simulink model "twolinkman"  (R2016a)
settings: Solver=VariableStepAuto  StartTime=0.0  StopTime=10.0  RelTol=1e-4
libraries: simulink x2
settings Model: Creator=Aniket  LastModifiedBy=Aniket

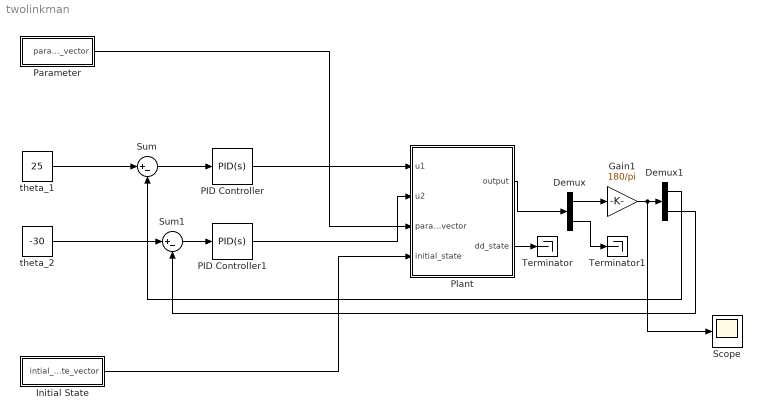
== system twolinkman ==
  Demux : Demux  Outputs=2
  Demux1 : Demux  Outputs=2
  Gain1 : Gain  Gain=180/pi
  Initial State : Subsystem
  PID Controller : simulink/Continuous/PID Controller  Controller=PID  TimeDomain=Continuous-time  SampleTime=-1  IntegratorMethod=Forward Euler  FilterMethod=Forward Euler  Form=Parallel  UseFilter=on  ControllerParametersSource=internal  P=0.928591865622313  I=0.934551024650747  D=0.226303191956831  N=743.239327840978  InitialConditionSource=internal  InitialConditionForIntegrator=0  InitialConditionForFilter=0  ExternalReset=none  LimitOutput=off  UpperSaturationLimit=inf  LowerSaturationLimit=-inf  LinearizeAsGain=on  AntiWindupMode=none  Kb=1  TrackingMode=off  Kt=1  PParamMin=[]  PParamMax=[]  IParamMin=[]  IParamMax=[]  DParamMin=[]  DParamMax=[]  NParamMin=[]  NParamMax=[]  KbParamMin=[]  KbParamMax=[]  KtParamMin=[]  KtParamMax=[]  POutMin=[]  POutMax=[]  IOutMin=[]  IOutMax=[]  DOutMin=[]  DOutMax=[]  NOutMin=[]  NOutMax=[]  KbOutMin=[]  KbOutMax=[]  KtOutMin=[]  KtOutMax=[]  IntegratorOutMin=[]  IntegratorOutMax=[]  FilterOutMin=[]  FilterOutMax=[]  SumOutMin=[]  SumOutMax=[]  SumI1OutMin=[]  SumI1OutMax=[]  SumI2OutMin=[]  SumI2OutMax=[]  SumI3OutMin=[]  SumI3OutMax=[]  SumDOutMin=[]  SumDOutMax=[]  SaturationOutMin=[]  SaturationOutMax=[]  IntegratorContinuousStateAttributes=''  IntegratorStateMustResolveToSignalObject=off  IntegratorRTWStateStorageClass=Auto  FilterContinuousStateAttributes=''  FilterStateMustResolveToSignalObject=off  FilterRTWStateStorageClass=Auto  DifferentiatorICPrevScaledInput=0  DifferentiatorOutMin=[]  DifferentiatorOutMax=[]
  PID Controller1 : simulink/Continuous/PID Controller  Controller=PID  TimeDomain=Continuous-time  SampleTime=-1  IntegratorMethod=Forward Euler  FilterMethod=Forward Euler  Form=Parallel  UseFilter=on  ControllerParametersSource=internal  P=3.82918167781898  I=9.14930088403733  D=0.205650241629809  N=18927.6604658624  InitialConditionSource=internal  InitialConditionForIntegrator=0  InitialConditionForFilter=0  ExternalReset=none  LimitOutput=off  UpperSaturationLimit=inf  LowerSaturationLimit=-inf  LinearizeAsGain=on  AntiWindupMode=none  Kb=1  TrackingMode=off  Kt=1  PParamMin=[]  PParamMax=[]  IParamMin=[]  IParamMax=[]  DParamMin=[]  DParamMax=[]  NParamMin=[]  NParamMax=[]  KbParamMin=[]  KbParamMax=[]  KtParamMin=[]  KtParamMax=[]  POutMin=[]  POutMax=[]  IOutMin=[]  IOutMax=[]  DOutMin=[]  DOutMax=[]  NOutMin=[]  NOutMax=[]  KbOutMin=[]  KbOutMax=[]  KtOutMin=[]  KtOutMax=[]  IntegratorOutMin=[]  IntegratorOutMax=[]  FilterOutMin=[]  FilterOutMax=[]  SumOutMin=[]  SumOutMax=[]  SumI1OutMin=[]  SumI1OutMax=[]  SumI2OutMin=[]  SumI2OutMax=[]  SumI3OutMin=[]  SumI3OutMax=[]  SumDOutMin=[]  SumDOutMax=[]  SaturationOutMin=[]  SaturationOutMax=[]  IntegratorContinuousStateAttributes=''  IntegratorStateMustResolveToSignalObject=off  IntegratorRTWStateStorageClass=Auto  FilterContinuousStateAttributes=''  FilterStateMustResolveToSignalObject=off  FilterRTWStateStorageClass=Auto  DifferentiatorICPrevScaledInput=0  DifferentiatorOutMin=[]  DifferentiatorOutMax=[]
  Parameter : Subsystem
  Plant : Subsystem
  Scope : Scope
  Sum : Sum  Inputs=|+-
  Sum1 : Sum  Inputs=|+-
  Terminator : Terminator
  Terminator1 : Terminator
  theta_1 : Constant  Value=25
  theta_2 : Constant  Value=-30
  wires:
  Plant/1(output) -> Demux/1
  Demux/1 -> Gain1/1
  theta_1/1 -> Sum/1
  theta_2/1 -> Sum1/1
  Sum/1 -> PID Controller/1
  PID Controller/1 -> Plant/1(u1)
  PID Controller1/1 -> Plant/2(u2)
  Sum1/1 -> PID Controller1/1
  Gain1/1 -> Scope/1, Demux1/1
  Demux1/1 -> Sum/2
  Demux1/2 -> Sum1/2
  Parameter/1("param_vector ") -> Plant/3(param_vector)
  Initial State/1(intial_state_vector) -> Plant/4(initial_state)
  Plant/2(dd_state) -> Terminator/1
  Demux/2 -> Terminator1/1

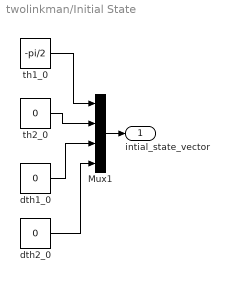
== system twolinkman/Initial State ==
  Mux1 : Mux
  dth1_0 : Constant  Value=0
  dth2_0 : Constant  Value=0
  th1_0 : Constant  Value=-pi/2
  th2_0 : Constant  Value=0
  intial_state_vector : Outport
  wires:
  Mux1/1 -> intial_state_vector/1
  dth2_0/1 -> Mux1/4
  th1_0/1 -> Mux1/1
  dth1_0/1 -> Mux1/3
  th2_0/1 -> Mux1/2

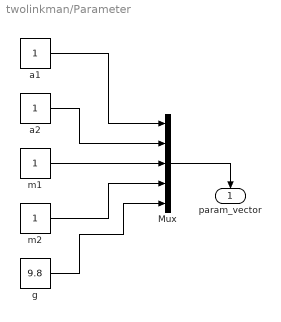
== system twolinkman/Parameter ==
  Mux : Mux  Inputs=5
  "a1 " : Constant
  a2 : Constant
  g : Constant  Value=9.8
  m1 : Constant
  m2 : Constant
  "param_vector " : Outport
  wires:
  m1/1 -> Mux/3
  Mux/1 -> "param_vector "/1
  g/1 -> Mux/5
  "a1 "/1 -> Mux/1
  m2/1 -> Mux/4
  a2/1 -> Mux/2

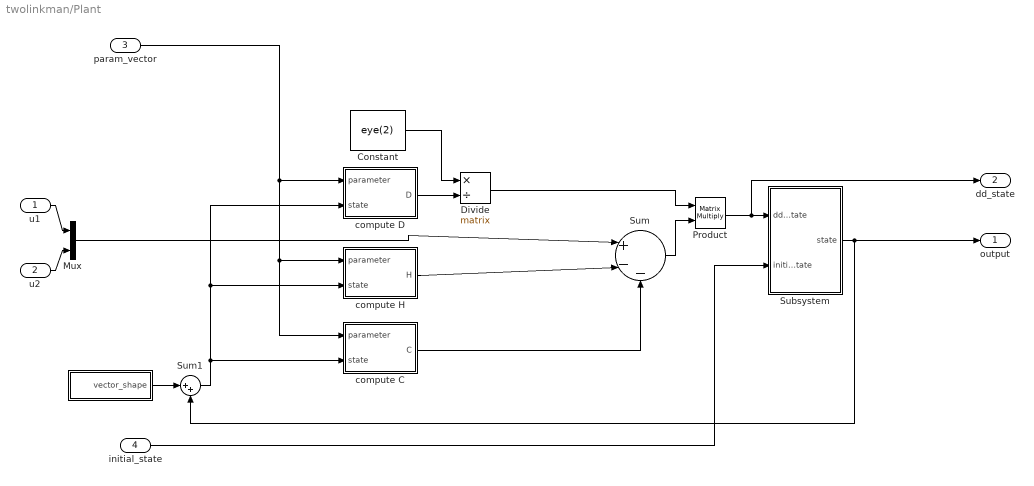
== system twolinkman/Plant ==
  u1 : Inport
  u2 : Inport  Port=2
  param_vector : Inport  Port=3
  initial_state : Inport  Port=4
  "  " : Subsystem
  Constant : Constant  Value=eye(2)
  Divide : Product  Inputs=*/  Multiplication=Matrix(*)
  Mux : Mux  Inputs=2
  Product : Product  Multiplication=Matrix(*)
  Subsystem : Subsystem
  Sum : Sum  Inputs=|+--
  Sum1 : Sum  Inputs=|++
  compute C : MATLAB Function  TreatAsAtomicUnit=on
  compute D : MATLAB Function  TreatAsAtomicUnit=on
  compute H : MATLAB Function  TreatAsAtomicUnit=on
  output : Outport
  dd_state : Outport  Port=2
  wires:
  Sum/1 -> Product/2
  compute C/1(C) -> Sum/3
  Constant/1 -> Divide/1
  initial_state/1 -> Subsystem/2(initial_state)
  compute H/1(H) -> Sum/2
  compute D/1(D) -> Divide/2
  Mux/1 -> Sum/1
  param_vector/1 -> compute C/1(parameter), compute H/1(parameter), compute D/1(parameter)
  Product/1 -> dd_state/1, Subsystem/1(dd_state)
  Sum1/1 -> compute D/2(state), compute H/2(state), compute C/2(state)
  "  "/1(vector_shape) -> Sum1/1
  Divide/1 -> Product/1
  u1/1 -> Mux/1
  Subsystem/1(state) -> output/1, Sum1/2
  u2/1 -> Mux/2

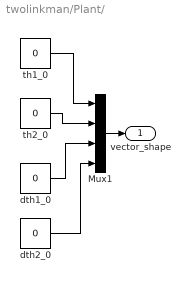
== system twolinkman/Plant/   ==
  Mux1 : Mux
  dth1_0 : Constant  Value=0
  dth2_0 : Constant  Value=0
  th1_0 : Constant  Value=0
  th2_0 : Constant  Value=0
  vector_shape : Outport
  wires:
  th2_0/1 -> Mux1/2
  dth1_0/1 -> Mux1/3
  th1_0/1 -> Mux1/1
  dth2_0/1 -> Mux1/4
  Mux1/1 -> vector_shape/1

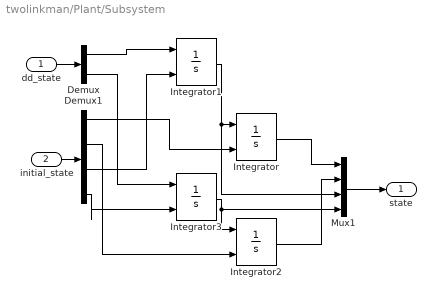
== system twolinkman/Plant/Subsystem ==
  dd_state : Inport
  initial_state : Inport  Port=2
  Demux : Demux  Outputs=2
  Demux1 : Demux
  Integrator{,1..3} (4 alike) : Integrator  InitialConditionSource=external
  Mux1 : Mux
  state : Outport
  wires:
  initial_state/1 -> Demux1/1
  dd_state/1 -> Demux/1
  Integrator/1 -> Mux1/1
  Integrator2/1 -> Mux1/2
  Demux/1 -> Integrator1/1
  Demux/2 -> Integrator3/1
  Integrator1/1 -> Mux1/3, Integrator/1
  Integrator3/1 -> Mux1/4, Integrator2/1
  Demux1/3 -> Integrator1/2
  Demux1/4 -> Integrator3/2
  Mux1/1 -> state/1
  Demux1/2 -> Integrator2/2
  Demux1/1 -> Integrator/2

== matlab function twolinkman/Plant/compute H ==
  data: parameter input; H output; state input
function H = H(parameter,state)
a1 = parameter(1);
a2 = parameter(2);
m1 = parameter(3);
m2 = parameter(4);
g = parameter(5);

if isempty(state)
    th1 = 0;
    th2 = 0;
    thd1 = 0;
    thd2 = 0;
else
    th1 = state(1);
    th2 = state(2);
    thd1 = state(3);
    thd2 = state(4);
end
H = [ -(a1*a2*m2*thd2*sin(th2)*(2*thd1 + thd2))/2;
                (a1*a2*m2*thd1^2*sin(th2))/2];

== matlab function twolinkman/Plant/compute D ==
  data: parameter input; D output; state input
function D = D(parameter,state)
a1 = parameter(1);
a2 = parameter(2);
m1 = parameter(3);
m2 = parameter(4);
g = parameter(5);

if isempty(state)
    th1 = 0;
    th2 = 0;
    thd1 = 0;
    thd2 = 0;
else
    th1 = state(1);
    th2 = state(2);
    thd1 = state(3);
    thd2 = state(4);
end

D = [ (a1^2*m1)/3 + a1^2*m2 + (a2^2*m2)/3 + a1*a2*m2*cos(th2), (a2*m2*(2*a2 + 3*a1*cos(th2)))/6;
    (a2*m2*(2*a2 + 3*a1*cos(th2)))/6,                      (a2^2*m2)/3];

== matlab function twolinkman/Plant/compute C ==
  data: parameter input; C output; state input
function C = C(parameter,state)
a1 = parameter(1);
a2 = parameter(2);
m1 = parameter(3);
m2 = parameter(4);
g = parameter(5);
if isempty(state)
    th1 = 0;
    th2 = 0;
    thd1 = 0;
    thd2 = 0;
else
    th1 = state(1);
    th2 = state(2);
    thd1 = state(3);
    thd2 = state(4);
end
C = [(g*(a1*m1*cos(th1) + 2*a1*m2*cos(th1) + a2*m2*cos(th1 + th2)))/2;
                                       (a2*g*m2*cos(th1 + th2))/2];
